simulink model "hdv_hydroelectropowertrain_model"  (R2026a)
settings: Solver=ode1be  StopTime=simulation_length  FixedStep=tsample  MaxStep=tsample
undefined symbols (not defined in the file): alpha, Apump, available_torque, Bpump, btheta_shaft, C1, consumption, Cpump, dp_lim, E0, E1, E2, E3, E_1, Elog, eta_v_m, eta_v_p, ki_dp_comp, ki_te_comp, kp_ctrl_m, kp_dp_comp, kp_te_comp, Kpump, load_blade_enable, Lpump, M, magnitude, Ncell, Npump, omega_e_rpm_ref, omega_l_max_rpm, q1Kalman, q2Kalman, q3Kalman, Qhr, R0, R1, R_tg, rKalman, rpm_base, rpm_consumption, simulation_length, tau_load, tau_load_max, Tc, torque_base, torque_consumption, torque_friction_base, tsample, v_track1_ref, v_track2_ref, valve_mmorifice_max, xv_m_max
libraries: fl_lib x383, nesl_utility x162, linear_swashplate_ctrl_lib x8, flexshaft_lib x5, bichamber_piston_lib x5, variable_displacement_motor_lib x4, variable_displacement_pump_lib x4, fixed_displacement_pump_lib x4, relief_valve_lib x4, inverse_shuttle_valve_lib x4, hydrostatic_threeway_valve_bichamber_piston_lib x4, hydrostatic_fourway_valve_bichamber_piston_lib x4
(part 8 of 8)

== matlab function hdv_hydroelectropowertrain_model/PR776_powertrain/electrical_main_drive_train/battery_management/kalman_observer_gains ==
  data: iz input; ts input; l1 output; z input; q1 input; q2 input; q3 input; r input; Qhr input; l2 output; l3 output
function [l1,l2,l3] = EKF(iz,ts,z,q1,q2,q3,r,Qhr)

    persistent  p11 p12 p13 p21 p22 p23 p31 p32 p33

    if isempty(p11)
        p11 = q1;
        p12 = 0;
        p13 = 0;
        p21 = 0;
        p22 = q2;
        p23 = 0;
        p31 = 0;
        p32 = 0;
        p33 = q3;
    end
    R = 0.015;
    C = 10;
    M = 125;
    E_1 = -1.031;
    E1 = 0.2156;
    E2 = 0;
    E3 = 0;
    Elog = -0.05;
    alpha = 35;
    Q = Qhr*3600;

    a11 = 1;
    a12 = 0;
    a13 = 0;
    a21 = 0;
    a22 = exp(-ts/(R*C));
    a23 = 0;
    a31 = 0;
    a32 = 0;
    a33 = abs(exp(-iz*ts/Q));

    c1 = -alpha*E_1*abs(exp(-alpha*z)) + E1 + 2*E2*z + 3*E3*z^2 - Elog/(1-z+ts);
    c2 = -R;
    c3 = M;
    
    p11_pr = a11*(a11*p11 + a12*p21 + a13*p31) + a12*(a11*p12 + a12*p22 + a13*p32) + a13*(a11*p13 + a12*p23 + a13*p33) + q1;

    p12_pr = a21*(a11*p11 + a12*p21 + a13*p31) + a22*(a11*p12 + a12*p22 + a13*p32) + a23*(a11*p13 + a12*p23 + a13*p33);

    p13_pr = a31*(a11*p11 + a12*p21 + a13*p31) + a32*(a11*p12 + a12*p22 + a13*p32) + a33*(a11*p13 + a12*p23 + a13*p33);

    p21_pr = a11*(a21*p11 + a22*p21 + a23*p31) + a12*(a21*p12 + a22*p22 + a23*p32) + a13*(a21*p13 + a22*p23 + a23*p33);

    p22_pr = a21*(a21*p11 + a22*p21 + a23*p31) + a22*(a21*p12 + a22*p22 + a23*p32) + a23*(a21*p13 + a22*p23 + a23*p33) + q2;

    p23_pr = a31*(a21*p11 + a22*p21 + a23*p31) + a32*(a21*p12 + a22*p22 + a23*p32) + a33*(a21*p13 + a22*p23 + a23*p33);

    p31_pr = a11*(a31*p11 + a32*p21 + a33*p31) + a12*(a31*p12 + a32*p22 + a33*p32) + a13*(a31*p13 + a32*p23 + a33*p33);

    p32_pr = a21*(a31*p11 + a32*p21 + a33*p31) + a22*(a31*p12 + a32*p22 + a33*p32) + a23*(a31*p13 + a32*p23 + a33*p33);

    p33_pr = a31*(a31*p11 + a32*p21 + a33*p31) + a32*(a31*p12 + a32*p22 + a33*p32) + a33*(a31*p13 + a32*p23 + a33*p33) + q3;

    den = c1*(c1*p11 + c2*p21 + c3*p31) + c2*(c1*p12 + c2*p22 + c3*p32) + c3*(c1*p13 + c2*p23 + c3*p33) + r;
 
    l1 = (c1*p11 + c2*p12 + c3*p13)/den;
    l2 = (c1*p21 + c2*p22 + c3*p23)/den;
    l3 = (c1*p31 + c2*p32 + c3*p33)/den;
    
    p11 = (1 - c1*l1)*p11_pr - c2*l1*p21_pr - c3*l1*p31_pr;
    
    p12 = (1 - c1*l1)*p12_pr - c2*l1*p22_pr - c3*l1*p32_pr;
    
    p13 = (1 - c1*l1)*p13_pr - c2*l1*p23_pr - c3*l1*p33_pr;
    
    p21 = -c1*l2*p11_pr + (1 - c2*l2)*p21_pr - c3*l2*p31_pr;
    
    p22 = -c1*l2*p12_pr + (1 - c2*l2)*p22_pr - c3*l2*p32_pr;
    
    p23 = -c1*l2*p13_pr + (1 - c2*l2)*p23_pr - c3*l2*p33_pr;
    
    p31 = -c1*l3*p11_pr - c2*l3*p21_pr + (1 - c3*l3)*p31_pr;
    
    p32 = -c1*l3*p12_pr - c2*l3*p22_pr + (1 - c3*l3)*p32_pr;
    
    p33 = -c1*l3*p13_pr - c2*l3*p23_pr + (1 - c3*l3)*p33_pr;
end

== matlab function hdv_hydroelectropowertrain_model/Vehicle Control System/feedforwards/Volumetric displacements calculation ==
  data: omega_e_rpm_ref input; Vd_p_R output; v_track1_ref input; v_track2_ref input; eta_vol_pump_right input; eta_vol_pump_left input; eta_vol_motor_right input; eta_vol_motor_left input; Vd_p_L output; v_track1_ref_cond output; v_track2_ref_cond output
function [Vd_p_R, Vd_p_L, v_track1_ref_cond, v_track2_ref_cond] = fcn(omega_e_rpm_ref, v_track1_ref, v_track2_ref, eta_vol_pump_right, eta_vol_pump_left, eta_vol_motor_right, eta_vol_motor_left)

n_tg = 54.31;
R_tg = 1.16/2;
Vm_nom = 280*2;
Vp_nom = 210*2;
v_track_sum_max = 18;
v_track_diff_max = 4;

eta_vol_tot_right = eta_vol_pump_right*eta_vol_motor_right;
eta_vol_tot_left = eta_vol_pump_left*eta_vol_motor_left;

v_track_sum = v_track1_ref + v_track2_ref;
v_track_diff = v_track1_ref - v_track2_ref;

if v_track_sum >= v_track_sum_max
    v_track_sum = v_track_sum_max;
end

if v_track_sum <= -v_track_sum_max
    v_track_sum = -v_track_sum_max;
end

if v_track_diff >= v_track_diff_max
    v_track_diff = v_track_diff_max;
end

if v_track_diff <= -v_track_diff_max
    v_track_diff = -v_track_diff_max;
end

v_track1_ref_cond = 1/2*(v_track_sum + v_track_diff);
v_track2_ref_cond = 1/2*(v_track_sum - v_track_diff);

omega_l_1_ref_rpm = v_track1_ref_cond/3.6/R_tg/(2*pi)*60;
omega_l_2_ref_rpm = v_track2_ref_cond/3.6/R_tg/(2*pi)*60;

d1_ff_temp = abs(Vm_nom/Vp_nom/eta_vol_tot_right*omega_l_1_ref_rpm/omega_e_rpm_ref*n_tg);
d2_ff_temp = abs(Vm_nom/Vp_nom/eta_vol_tot_left*omega_l_2_ref_rpm/omega_e_rpm_ref*n_tg);

if d1_ff_temp >= 1
    Vd_p_R = 2 - 1/d1_ff_temp;
else
    Vd_p_R = d1_ff_temp;
end
if d2_ff_temp >= 1
    Vd_p_L = 2 - 1/d2_ff_temp;
else
    Vd_p_L = d2_ff_temp;
end

== matlab function hdv_hydroelectropowertrain_model/PR776_powertrain/electrical_main_drive_train/battery_management/lithium-ion battery model ==
  data: iz input; SOC output; u output; ts input; Qhr input; l1 input; l2 input; l3 input; vout input; x output
function [SOC, u, x] = lithium_ion_battery(iz,ts,Qhr,l1,l2,l3,vout)

    persistent z_po ir_po h_po vout_hat

    if isempty(z_po)
        ir_po = 0;
        h_po = 0;
        z_po = 0;        
    end
    
        R0 = 0.015;
        R = 0.015;
        C = 10;
        M = 125;
        E_1 = -1.031;
        E0 = 3.685;
        E1 = 0.2156;
        E2 = 0;
        E3 = 0;
        Elog = -0.05;
        alpha = 35;
        N = 185;
        Q = Qhr*3600;
        
        
        if z_po > 1
            z_pr = z_po;
        elseif z_po < 0
            z_pr = z_po;
        else
            z_pr = z_po - ts/Q*iz ;
        end
        ir_pr = exp(-ts/(R*C))*ir_po + (1-exp(-ts/(R*C)))*iz;

        h_pr = exp(-abs(iz)*ts/Q)*h_po - (1-exp(-abs(iz)*ts/Q))*sign(iz);
        
        OCV = E_1*exp(-z_pr*alpha) + E0 + E1*z_pr + E2*z_pr^2 + E3*z_pr^3 + Elog * log(abs(1-z_pr+ts));
        
        vout_hat = OCV*N + M*h_pr - R*ir_pr - R0*iz;
        
        z_po = z_pr + l1*(vout - vout_hat);
        ir_po = ir_pr + l2*(vout - vout_hat);
        h_po = h_pr + l3*(vout - vout_hat);
        u = vout_hat;
        
        x = [z_po; ir_po; h_po];

    SOC = z_po;
end
